simulink model "MIMO_FIXED"  (R2017a)
settings: Solver=VariableStepAuto  StartTime=0.0  StopTime=1000  RelTol=1e-3
libraries: dspsigops x80, commchan3 x4, commdigbbndpm3 x2, commfilt2 x2, commsink2 x1, commutil2 x1
(part 6 of 6)

== system MIMO_FIXED/Transceiver7/Interpolation 1/comb_filter/E1 ==
  In1 : Inport
  Data Type Conversion1 : DataTypeConversion  OutDataTypeStr=fixdt(1,19,0)  SaturateOnIntegerOverflow=on
  Data Type Conversion2 : DataTypeConversion  OutDataTypeStr=fixdt(1,19,0)  SaturateOnIntegerOverflow=on
  Data Type Conversion3 : DataTypeConversion  OutDataTypeStr=fixdt(1,13,0)  SaturateOnIntegerOverflow=on
  Data Type Conversion4 : DataTypeConversion  OutDataTypeStr=fixdt(1,19,0)  SaturateOnIntegerOverflow=on
  Data Type Conversion5 : DataTypeConversion  OutDataTypeStr=fixdt(1,20,0)  SaturateOnIntegerOverflow=on
  Data Type Conversion7 : DataTypeConversion  OutDataTypeStr=fixdt(1,15,0)  SaturateOnIntegerOverflow=on
  Delay3 : Delay  DelayLength=1
  Delay4 : Delay  DelayLength=1
  Delay5 : Delay  DelayLength=1
  Gain : Gain  Gain=20
  Gain1 : Gain  Gain=284
  Gain2 : Gain  Gain=204
  Gain3 : Gain  Gain=4
  Sum : Sum
  Sum1 : Sum
  Sum2 : Sum
  Out1 : Outport
  wires:
  Sum/1 -> Data Type Conversion4/1
  Delay3/1 -> Sum/2
  Delay4/1 -> Sum1/2
  Delay5/1 -> Sum2/2
  Gain/1 -> Data Type Conversion7/1
  Data Type Conversion7/1 -> Delay3/1
  Gain1/1 -> Data Type Conversion1/1
  Data Type Conversion1/1 -> Sum/1
  Gain2/1 -> Data Type Conversion2/1
  Data Type Conversion2/1 -> Sum1/1
  Gain3/1 -> Data Type Conversion3/1
  Data Type Conversion3/1 -> Sum2/1
  Data Type Conversion4/1 -> Delay4/1
  Sum1/1 -> Data Type Conversion5/1
  Data Type Conversion5/1 -> Delay5/1
  In1/1 -> Gain2/1, Gain3/1, Gain1/1, Gain/1
  Sum2/1 -> Out1/1

== system MIMO_FIXED/Transceiver7/Interpolation 1/comb_filter/E2 ==
  In1 : Inport
  Data Type Conversion : DataTypeConversion  OutDataTypeStr=fixdt(1,14,0)
  Data Type Conversion1 : DataTypeConversion  OutDataTypeStr=fixdt(1,19,0)
  Data Type Conversion2 : DataTypeConversion  OutDataTypeStr=fixdt(1,19,0)
  Data Type Conversion3 : DataTypeConversion  OutDataTypeStr=fixdt(1,20,0)
  Delay3 : Delay  DelayLength=1
  Delay4 : Delay  DelayLength=1
  Delay5 : Delay  DelayLength=1
  Gain : Gain  Gain=10
  Gain1 : Gain  Gain=246
  Sum : Sum
  Sum1 : Sum
  Sum2 : Sum
  Out1 : Outport
  wires:
  Sum1/1 -> Data Type Conversion3/1
  Delay3/1 -> Sum/2
  Delay4/1 -> Sum1/2
  Delay5/1 -> Sum2/2
  Data Type Conversion/1 -> Delay3/1, Sum2/1
  Gain/1 -> Data Type Conversion/1
  Gain1/1 -> Data Type Conversion1/1
  Data Type Conversion1/1 -> Sum1/1, Sum/1
  Data Type Conversion2/1 -> Delay4/1
  Sum/1 -> Data Type Conversion2/1
  Data Type Conversion3/1 -> Delay5/1
  In1/1 -> Gain1/1, Gain/1
  Sum2/1 -> Out1/1

== system MIMO_FIXED/Transceiver7/Interpolation 1/comb_filter/E3 ==
  In1 : Inport
  Data Type Conversion : DataTypeConversion  OutDataTypeStr=fixdt(1,13,0)
  Data Type Conversion1 : DataTypeConversion  OutDataTypeStr=fixdt(1,19,0)
  Data Type Conversion2 : DataTypeConversion  OutDataTypeStr=fixdt(1,19,0)
  Data Type Conversion3 : DataTypeConversion  OutDataTypeStr=fixdt(1,15,0)
  Data Type Conversion4 : DataTypeConversion  OutDataTypeStr=fixdt(1,19,0)
  Data Type Conversion5 : DataTypeConversion  OutDataTypeStr=fixdt(1,20,0)
  Delay3 : Delay  DelayLength=1
  Delay4 : Delay  DelayLength=1
  Delay5 : Delay  DelayLength=1
  Gain : Gain  Gain=4
  Gain1 : Gain  Gain=204
  Gain2 : Gain  Gain=284
  Gain3 : Gain  Gain=20
  Sum : Sum
  Sum1 : Sum
  Sum2 : Sum
  Out1 : Outport
  wires:
  Delay3/1 -> Sum/2
  Delay4/1 -> Sum1/2
  Delay5/1 -> Sum2/2
  Gain/1 -> Data Type Conversion/1
  Data Type Conversion/1 -> Delay3/1
  Gain1/1 -> Data Type Conversion1/1
  Data Type Conversion1/1 -> Sum/1
  Gain2/1 -> Data Type Conversion2/1
  Data Type Conversion2/1 -> Sum1/1
  Gain3/1 -> Data Type Conversion3/1
  Data Type Conversion3/1 -> Sum2/1
  Sum/1 -> Data Type Conversion4/1
  Data Type Conversion4/1 -> Delay4/1
  Sum1/1 -> Data Type Conversion5/1
  Data Type Conversion5/1 -> Delay5/1
  Sum2/1 -> Out1/1
  In1/1 -> Gain3/1, Gain2/1, Gain1/1, Gain/1

== system MIMO_FIXED/Transceiver7/Interpolation 1/comb_filter/E4 ==
  In1 : Inport
  Data Type Conversion1 : DataTypeConversion  OutDataTypeStr=fixdt(1,18,0)  SaturateOnIntegerOverflow=on
  Data Type Conversion12 : DataTypeConversion  OutDataTypeStr=fixdt(1,11,0)  SaturateOnIntegerOverflow=on
  Data Type Conversion2 : DataTypeConversion  OutDataTypeStr=fixdt(1,19,0)  SaturateOnIntegerOverflow=on
  Data Type Conversion3 : DataTypeConversion  OutDataTypeStr=fixdt(1,16,0)  SaturateOnIntegerOverflow=on
  Data Type Conversion4 : DataTypeConversion  OutDataTypeStr=fixdt(1,18,0)  SaturateOnIntegerOverflow=on
  Data Type Conversion5 : DataTypeConversion  OutDataTypeStr=fixdt(1,19,0)  SaturateOnIntegerOverflow=on
  Delay3 : Delay  DelayLength=1
  Delay4 : Delay  DelayLength=1
  Delay5 : Delay  DelayLength=1
  Gain : Gain
  Gain1 : Gain  Gain=161
  Gain2 : Gain  Gain=315
  Gain3 : Gain  Gain=35
  Sum : Sum
  Sum1 : Sum
  Sum2 : Sum
  Out1 : Outport
  wires:
  Sum1/1 -> Data Type Conversion5/1
  Sum/1 -> Data Type Conversion4/1
  Gain1/1 -> Data Type Conversion1/1
  Delay3/1 -> Sum/2
  Delay4/1 -> Sum1/2
  Gain3/1 -> Data Type Conversion3/1
  Delay5/1 -> Sum2/2
  Gain/1 -> Data Type Conversion12/1
  Data Type Conversion12/1 -> Delay3/1
  Data Type Conversion1/1 -> Sum/1
  Gain2/1 -> Data Type Conversion2/1
  Data Type Conversion2/1 -> Sum1/1
  Data Type Conversion3/1 -> Sum2/1
  Data Type Conversion4/1 -> Delay4/1
  Data Type Conversion5/1 -> Delay5/1
  In1/1 -> Gain2/1, Gain3/1, Gain1/1, Gain/1
  Sum2/1 -> Out1/1

== system MIMO_FIXED/Transceiver7/Interpolation 1/comb_filter/E5 ==
  In1 : Inport
  Data Type Conversion1 : DataTypeConversion  OutDataTypeStr=fixdt(1,19,0)  SaturateOnIntegerOverflow=on
  Data Type Conversion12 : DataTypeConversion  OutDataTypeStr=fixdt(1,18,0)  SaturateOnIntegerOverflow=on
  Data Type Conversion2 : DataTypeConversion  OutDataTypeStr=fixdt(1,17,0)  SaturateOnIntegerOverflow=on
  Data Type Conversion3 : DataTypeConversion  OutDataTypeStr=fixdt(1,19,0)  SaturateOnIntegerOverflow=on
  Delay6 : Delay  DelayLength=1
  Delay7 : Delay  DelayLength=1
  Gain4 : Gain  Gain=120
  Gain5 : Gain  Gain=336
  Gain6 : Gain  Gain=56
  Sum4 : Sum
  Sum5 : Sum
  Out1 : Outport
  wires:
  Gain4/1 -> Data Type Conversion12/1
  Sum4/1 -> Data Type Conversion3/1
  Delay7/1 -> Sum5/2
  Gain6/1 -> Data Type Conversion2/1
  Delay6/1 -> Sum4/2
  Data Type Conversion12/1 -> Delay6/1
  Gain5/1 -> Data Type Conversion1/1
  Data Type Conversion1/1 -> Sum4/1
  Data Type Conversion2/1 -> Sum5/1
  Data Type Conversion3/1 -> Delay7/1
  In1/1 -> Gain6/1, Gain5/1, Gain4/1
  Sum5/1 -> Out1/1

== system MIMO_FIXED/Transceiver7/Interpolation 1/comb_filter/E6 ==
  In1 : Inport
  Data Type Conversion1 : DataTypeConversion  OutDataTypeStr=fixdt(1,20,0)  SaturateOnIntegerOverflow=on
  Data Type Conversion2 : DataTypeConversion  OutDataTypeStr=fixdt(1,20,0)  SaturateOnIntegerOverflow=on
  Data Type Conversion3 : DataTypeConversion  OutDataTypeStr=fixdt(1,17,0)  SaturateOnIntegerOverflow=on
  Delay6 : Delay  DelayLength=1
  Delay7 : Delay  DelayLength=1
  Gain4 : Gain  Gain=84
  Gain5 : Gain  Gain=344
  Sum4 : Sum
  Sum5 : Sum
  Out1 : Outport
  wires:
  Delay7/1 -> Sum5/2
  Gain4/1 -> Data Type Conversion3/1
  Gain5/1 -> Data Type Conversion1/1
  Delay6/1 -> Sum4/2
  Data Type Conversion3/1 -> Sum5/1, Delay6/1
  Data Type Conversion1/1 -> Sum4/1
  Sum4/1 -> Data Type Conversion2/1
  Data Type Conversion2/1 -> Delay7/1
  In1/1 -> Gain5/1, Gain4/1
  Sum5/1 -> Out1/1

== system MIMO_FIXED/Transceiver7/Interpolation 1/comb_filter/E7 ==
  In1 : Inport
  Data Type Conversion1 : DataTypeConversion  OutDataTypeStr=fixdt(1,19,0)  SaturateOnIntegerOverflow=on
  Data Type Conversion12 : DataTypeConversion  OutDataTypeStr=fixdt(1,17,0)  SaturateOnIntegerOverflow=on
  Data Type Conversion2 : DataTypeConversion  OutDataTypeStr=fixdt(1,18,0)  SaturateOnIntegerOverflow=on
  Data Type Conversion3 : DataTypeConversion  OutDataTypeStr=fixdt(1,19,0)  SaturateOnIntegerOverflow=on
  Delay6 : Delay  DelayLength=1
  Delay7 : Delay  DelayLength=1
  Gain4 : Gain  Gain=56
  Gain5 : Gain  Gain=336
  Gain6 : Gain  Gain=120
  Sum4 : Sum
  Sum5 : Sum
  Out1 : Outport
  wires:
  Gain4/1 -> Data Type Conversion12/1
  Sum4/1 -> Data Type Conversion3/1
  Delay7/1 -> Sum5/2
  Gain6/1 -> Data Type Conversion2/1
  Delay6/1 -> Sum4/2
  Data Type Conversion12/1 -> Delay6/1
  Gain5/1 -> Data Type Conversion1/1
  Data Type Conversion1/1 -> Sum4/1
  Data Type Conversion2/1 -> Sum5/1
  Data Type Conversion3/1 -> Delay7/1
  In1/1 -> Gain6/1, Gain5/1, Gain4/1
  Sum5/1 -> Out1/1
